simulink model "milestoneone_mdl_v2"  (R2025a)
settings: Solver=FixedStepAuto  StartTime=0.0  StopTime=10  FixedStep=1e-3  RelTol=1e-3  EnableMultiTasking=on
model workspace (MAT data in the model file):
  Var = 0
undefined symbols (not defined in the file): D0, D1, D10, D11, D12, D13, D2, D3, D4, D5, D6, D7, D8, D9, PTA0, PTA1, PTA2, PTB23, PTB9, PTC16, PTC17, PTC2, PTC3, PTC4, PTD0, PTD1, PTD2, PTD3
libraries: frdmk64flib x14
settings Model: ExtModeTrigDuration=5  Creator=alber  LastModifiedBy=ybakr
settings OptimizationCC: DefaultParameterBehavior=Inlined  EnhancedBackFolding=on  PassReuseOutputArgsAs=Individual arguments  ZeroExternalMemoryAtStartup=off  ZeroInternalMemoryAtStartup=off  MaxStackSize=64  OptimizeBlockOrder=speed  DifferentSizesBufferReuse=on  OptimizationCustomize=off  EfficientTunableParamExpr=on
settings DebuggingCC: ParameterTunabilityLossMsg=error
settings HardwareCC: ProdBitPerPointer=32.0  ProdBitPerSizeT=32.0  ProdBitPerPtrDiffT=32.0  ProdLargestAtomicInteger=Long  ProdLargestAtomicFloat=Double  ProdWordSize=32.0  ProdHWDeviceType=ARM Compatible->ARM Cortex
settings SFSimCC: MATLABDynamicMemAlloc=off
settings RTWCC: SystemTargetFile=ert.tlc  HardwareBoard=NXP FRDM-K64F  TLCOptions="-aInlineSetEventsForThisBaseRateFcn=TLC_FALSE -aSuppressMultiTaskScheduler=TLC_FALSE  -aRateBasedStepFcn=0"  TemplateMakefile=ert_default_tmf  Toolchain=GNU Tools for ARM Embedded Processors  Description=Embedded Coder
settings CodeAppCC: ForceParamTrailComments=on  IgnoreCustomStorageClasses=off  OperatorAnnotations=on  SimulinkDataObjDesc=on  SFDataObjDesc=on  InsertBlockDesc=on
settings ERTTargetCC: ExtModeTransport=4.0  ExtModeStaticAlloc=off  ExtModeMexFile=sendToCommService  ExtModeIntrfLevel=Level1

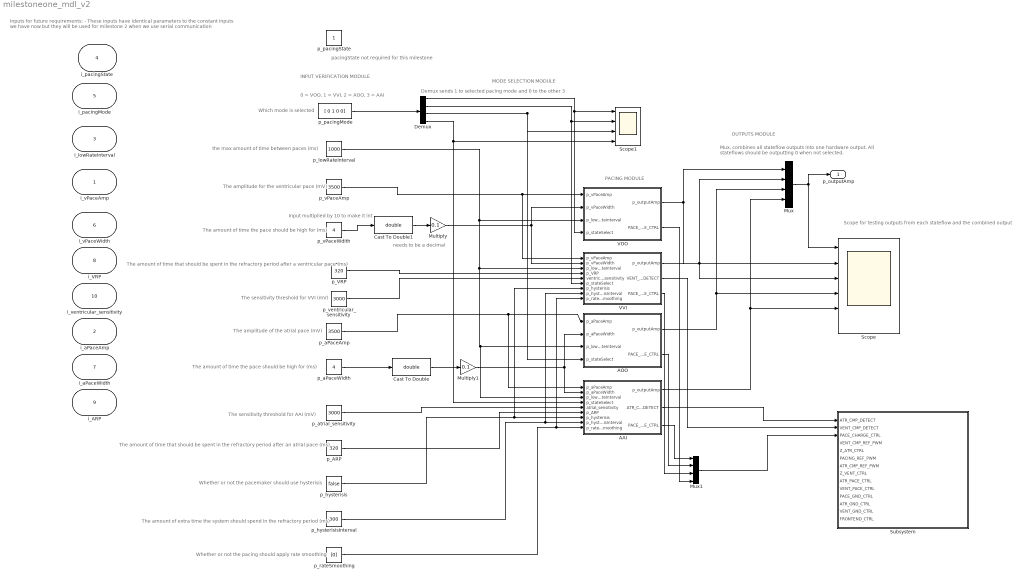
== system milestoneone_mdl_v2 ==
  note: The amount of extra time the system should spend in the refractory period (ms)
  note: Whether or not the pacemaker should use hysterisis
  note: Whether or not the pacing should apply rate smoothing
  note: The amplitude of the atrial pace (mV)
  note: The sensitivity threshold for VVI (mV)
  note: The amount of time that should be spent in the refractory period after a ventricular pace (ms)
  note: The amount of time the pace should be high for (ms)
  note: needs to be a decimal
  note: OUTPUTS MODULE
  note: PACING MODULE
  note: MODE SELECTION MODULE
  note: INPUT VERIFICATION MODULE
  note: The amplitude for the ventricular pace (mV)
  note: the max amount of time between paces (ms)
  note: Which mode is selected
  note: Inputs for future requirements:
      | - These inputs have identical parameters to the constant inputs we have now but they will be used for milestone 2 when we use serial communication
  note: pacingState not required for this milestone
  note: Demux sends 1 to selected pacing mode and 0 to the other 3
  note: Input multiplied by 10 to make it int
  note: 0 = VOO, 1 = VVI, 2 = AOO, 3 = AAI
  note: Scope for testing outputs from each stateflow and the combined output
  note: Mux, combines all stateflow outputs into one hardware output.
      | All stateflows should be outputting 0 when not selected.
  note: The amount of time the pace should be high for (ms)
  note: The sensitivity threshold for AAI (mV)
  note: The amount of time that should be spent in the refractory period after an atrial pace (ms)
  i_vPaceAmp : Inport  OutMin=[500]  OutMax=[7000]  OutDataTypeStr=uint16  Unit=mV  PortDimensions=1
  i_aPaceAmp : Inport  Port=2  OutMin=[500]  OutMax=[7000]  OutDataTypeStr=uint16  Unit=mV  PortDimensions=1
  i_lowRateInterval : Inport  Port=3  OutMin=[343]  OutMax=[2000]  OutDataTypeStr=uint16  Unit=Msec  PortDimensions=1
  i_pacingState : Inport  Port=4
  i_pacingMode : Inport  Port=5  OutDataTypeStr=uint8  PortDimensions=1
  i_vPaceWidth : Inport  Port=6  OutMin=1  OutMax=19  OutDataTypeStr=uint16  Unit=Msec  PortDimensions=1
  i_aPaceWidth : Inport  Port=7  OutMin=[1]  OutMax=[19]  OutDataTypeStr=uint16  Unit=Msec  PortDimensions=1
  i_VRP : Inport  Port=8  OutMin=[150]  OutMax=[500]  OutDataTypeStr=uint16  Unit=Msec  PortDimensions=1
  i_ARP : Inport  Port=9  OutMin=[150]  OutMax=[500]  OutDataTypeStr=uint16  Unit=mSec  PortDimensions=1
  i_ventricular_sensitivity : Inport  Port=10  OutDataTypeStr=uint16  PortDimensions=1
  AAI : Stateflow chart  TreatAsAtomicUnit=on
      settings: PortSchema="{\"entries\":[{\"content\":{\"sides\":[{\"content\":{\"connectorIds\":[\"In6\",\"In1\",\"In2\",\"In3\",\"In4\",\"In5\",\"In7\",\"In8\",\"In9\"]},\"type\":\"ConnectorPlacement.EquallySpacedRectSide\",\"uuid\":\"cccc9f32-b255-4089-8202-5f4b6cf4849a\"},{\"content\":{\"connectorIds\":[\"Out1\",\"Out2\",\"Out3\"],\"side\":\"RIGHT\"},\"type\":\"ConnectorPlacement.EquallySpacedRectSide\",\"uuid\":\"983a4a60-3d5c-4e53-84aa-b68c0bc6099e\"},{\"content\":{\"side\":\"TOP\"},\"type\":\"ConnectorPlacement.EquallySpacedRectSide\",\"uuid\":\"2756b790-cbb9-4039-b4f9-91cb14419ddd\"}]},\"type\":\"ConnectorPlacement.EquallySpacedConnector\",\"uuid\":\"1ccddf37-9dbc-46c0-8904-a3b9c6a38aa8\"}],\"packageUris\":[\"http://schema.mathworks.com/mf0/Connector/R2020b\"],\"version\":\"1.0\"}"
  AOO : Stateflow chart  TreatAsAtomicUnit=on
  Cast To Double : DataTypeConversion  OutDataTypeStr=double  SaturateOnIntegerOverflow=off  RndMeth=Floor
  Cast To Double1 : DataTypeConversion  OutDataTypeStr=double  SaturateOnIntegerOverflow=off  RndMeth=Floor
  Demux : Demux
  Multiply : Gain  Gain=0.1
  Multiply1 : Gain  Gain=0.1
  Mux : Mux
  Mux1 : Mux
  Scope : Scope  NumInputPorts=6
      settings: ActiveDisplayYMinimum=-128.4248  ActiveDisplayYMaximum=3655.0816
  Scope1 : Scope  NumInputPorts=4
      settings: ActiveDisplayYMinimum=-0.2183  ActiveDisplayYMaximum=1.8178
  Subsystem : Subsystem
  VOO : Stateflow chart  TreatAsAtomicUnit=on
  VVI : Stateflow chart  TreatAsAtomicUnit=on
  p_ARP : Constant  Value=320  OutMin=[150]  OutMax=[500]  OutDataTypeStr=uint16
  p_VRP : Constant  Value=320  OutMin=[150]  OutMax=[500]  OutDataTypeStr=uint16
  p_aPaceAmp : Constant  Value=3500  OutDataTypeStr=uint16
  p_aPaceWidth : Constant  Value=4  OutDataTypeStr=int16
  p_atrial_sensitivity : Constant  Value=3000  OutDataTypeStr=uint16
  p_hysterisis : Constant  Value=false  OutDataTypeStr=uint16
  p_hysterisisInterval : Constant  Value=300  OutDataTypeStr=uint16
  p_lowRateInterval : Constant  Value=1000  OutMin=[343]  OutMax=[2000]  OutDataTypeStr=uint16
  p_pacingMode : Constant  Value=[ 0 1 0 0]  OutDataTypeStr=uint8
  p_pacingState : Constant  OutDataTypeStr=uint8
  p_rateSmoothing : Constant  Value=[0]  OutDataTypeStr=uint16
  p_vPaceAmp : Constant  Value=3500  OutMin=[500]  OutMax=[7000]  OutDataTypeStr=uint16
  p_vPaceWdith : Constant  Value=4  OutMin=[1]  OutMax=[19]  OutDataTypeStr=int16
  p_ventricular_sensitivity : Constant  Value=3000  OutDataTypeStr=uint16
  p_outputAmp : Outport
  wires:
  VVI/1(p_outputAmp) -> Mux/2, Scope/3
  AOO/1(p_outputAmp) -> Mux/3, Scope/4
  Mux/1 -> p_outputAmp/1, Scope/1
  Multiply/1 -> VOO/2(p_vPaceWidth), VVI/2(p_vPaceWidth)
  Cast To Double1/1 -> Multiply/1
  Cast To Double/1 -> Multiply1/1
  Multiply1/1 -> AAI/1(p_aPaceWidth), AOO/2(p_aPaceWidth)
  Demux/1 -> Scope1/1, VOO/4(p_stateSelect)
  Demux/2 -> Scope1/2, VVI/6(p_stateSelect)
  Demux/3 -> Scope1/3, AOO/4(p_stateSelect)
  Demux/4 -> AAI/3(p_stateSelect), Scope1/4
  p_pacingMode/1 -> Demux/1
  p_aPaceWidth/1 -> Cast To Double/1
  p_aPaceAmp/1 -> AAI/6(p_aPaceAmp), AOO/1(p_aPaceAmp)
  p_lowRateInterval/1 -> AAI/2(p_lowRateInterval), AOO/3(p_lowRateInterval), VVI/3(p_lowRateInterval), VOO/3(p_lowRateInterval)
  p_vPaceAmp/1 -> VVI/1(p_vPaceAmp), VOO/1(p_vPaceAmp)
  p_vPaceWdith/1 -> Cast To Double1/1
  p_VRP/1 -> VVI/4(p_VRP)
  p_ventricular_sensitivity/1 -> VVI/5(ventricular_sensitivity)
  VOO/1(p_outputAmp) -> Scope/2, Mux/1
  p_ARP/1 -> AAI/5(p_ARP)
  p_atrial_sensitivity/1 -> AAI/4(atrial_sensitivity)
  p_hysterisis/1 -> VVI/7(p_hysterisis), AAI/7(p_hysterisis)
  p_hysterisisInterval/1 -> VVI/8(p_hysterisisInterval), AAI/8(p_hysterisisInterval)
  p_rateSmoothing/1 -> VVI/9(p_rateSmoothing), AAI/9(p_rateSmoothing)
  AAI/1(p_outputAmp) -> Mux/4, Scope/5
  AAI/2(ATR_CMP_DETECT) -> Subsystem/1("ATR_CMP_DETECT ")
  VVI/2(VENT_CMP_DETECT) -> Subsystem/2(VENT_CMP_DETECT)
  AAI/3(PACE_CHARGE_CTRL) -> Mux1/1
  Mux1/1 -> Subsystem/3(PACE_CHARGE_CTRL)
  AOO/2(PACE_CHARGE_CTRL) -> Mux1/2
  VVI/3(PACE_CHARGE_CTRL) -> Mux1/3
  VOO/2(PACE_CHARGE_CTRL) -> Mux1/4

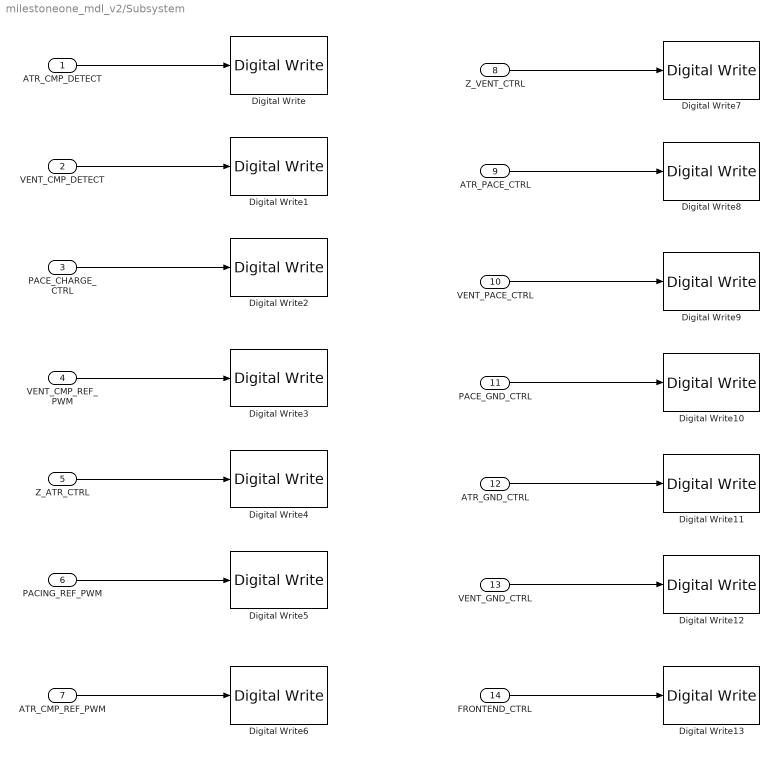
== system milestoneone_mdl_v2/Subsystem ==
  "ATR_CMP_DETECT " : Inport
  VENT_CMP_DETECT : Inport  Port=2
  PACE_CHARGE_CTRL : Inport  Port=3
  VENT_CMP_REF_PWM : Inport  Port=4
  Z_ATR_CTRL : Inport  Port=5
  PACING_REF_PWM : Inport  Port=6
  ATR_CMP_REF_PWM : Inport  Port=7
  Z_VENT_CTRL : Inport  Port=8
  ATR_PACE_CTRL : Inport  Port=9
  VENT_PACE_CTRL : Inport  Port=10
  PACE_GND_CTRL : Inport  Port=11
  ATR_GND_CTRL : Inport  Port=12
  VENT_GND_CTRL : Inport  Port=13
  FRONTEND_CTRL : Inport  Port=14
  Digital Write : frdmk64flib/Digital Write  Whichpin=PTC16 (D0)
  Digital Write1 : frdmk64flib/Digital Write  Whichpin=PTC17 (D1)
  Digital Write10 : frdmk64flib/Digital Write  Whichpin=PTD0 (D10)
  Digital Write11 : frdmk64flib/Digital Write  Whichpin=PTD2 (D11)
  Digital Write12 : frdmk64flib/Digital Write  Whichpin=PTD3 (D12)
  Digital Write13 : frdmk64flib/Digital Write  Whichpin=PTD1 (D13)
  Digital Write2 : frdmk64flib/Digital Write  Whichpin=PTB9 (D2)
  Digital Write3 : frdmk64flib/Digital Write  Whichpin=PTA1 (D3)
  Digital Write4 : frdmk64flib/Digital Write  Whichpin=PTB23 (D4)
  Digital Write5 : frdmk64flib/Digital Write  Whichpin=PTA2 (D5)
  Digital Write6 : frdmk64flib/Digital Write  Whichpin=PTC2 (D6)
  Digital Write7 : frdmk64flib/Digital Write  Whichpin=PTC3 (D7)
  Digital Write8 : frdmk64flib/Digital Write  Whichpin=PTA0 (D8)
  Digital Write9 : frdmk64flib/Digital Write  Whichpin=PTC4 (D9)
  wires:
  "ATR_CMP_DETECT "/1 -> Digital Write/1
  VENT_CMP_DETECT/1 -> Digital Write1/1
  PACE_CHARGE_CTRL/1 -> Digital Write2/1
  Z_ATR_CTRL/1 -> Digital Write4/1
  PACING_REF_PWM/1 -> Digital Write5/1
  VENT_CMP_REF_PWM/1 -> Digital Write3/1
  Z_VENT_CTRL/1 -> Digital Write7/1
  PACE_GND_CTRL/1 -> Digital Write10/1
  ATR_GND_CTRL/1 -> Digital Write11/1
  ATR_PACE_CTRL/1 -> Digital Write8/1
  VENT_PACE_CTRL/1 -> Digital Write9/1
  ATR_CMP_REF_PWM/1 -> Digital Write6/1
  VENT_GND_CTRL/1 -> Digital Write12/1
  FRONTEND_CTRL/1 -> Digital Write13/1

== stateflow chart milestoneone_mdl_v2/AOO ==
  note: Max total cycle time - time already elapsed this cycle
  note: AOO Pacing Mode
  note: Cycle through this state when AoO isn't selected
  state PACE
    entry:
    %Send out pace signal
    p_outputAmp = p_aPaceAmp;
    current_state = "AOO PACE"
    PACE_CHARGE_CTRL = 0;
    % Wait for the width of a pace
  state CHARGE
    entry:
    % Stop pacing, wait rest of cycle time
    p_outputAmp = 0;
    current_state = "AOO CHARGE"
    PACE_CHARGE_CTRL = 1;
  state INACTIVE
    % When state is not selected by input
  CHARGE -> PACE [order 2] : [after(p_lowRateInterval - p_aPaceWidth, msec)]
  (default) -> INACTIVE
  INACTIVE -> CHARGE [order 1] : [p_stateSelect == 1]
  CHARGE -> INACTIVE [order 1] : [p_stateSelect == 0]
  INACTIVE -> INACTIVE [order 2] : [p_stateSelect == 0]
  PACE -> CHARGE : after(p_aPaceWidth, msec)
  data: data local; p_outputAmp output uint16; p_aPaceAmp input uint16 =3500; p_aPaceWidth input double =0.4; p_lowRateInterval input uint16 =6000/low_rate_lim; p_stateSelect input uint8; current_state local string; PACE_CHARGE_CTRL output

== stateflow chart milestoneone_mdl_v2/VOO ==
  note: Total cycle time - time already elapsed this cycle
  note: VOO Pacing Mode
  state CHARGE
    entry:
    % Output 0V
    p_outputAmp = 0;
    current_state = "VOO CHARGE"
    PACE_CHARGE_CTRL = 1;
    % Rest time = total cycle time - pace width
  state PACE
    entry:
    % Output pace at specified amplitude
    p_outputAmp = p_vPaceAmp;
    current_state = "VOO PACE"
    PACE_CHARGE_CTRL = 0;
    % Wait so that the pace has the specified width
  state INACTIVE
    % Stateflow is inactive when not selected
  CHARGE -> PACE [order 2] : [after(p_lowRateInterval - p_vPaceWidth, msec)]
  (default) -> INACTIVE
  INACTIVE -> CHARGE [order 1] : [p_stateSelect == 1]
  CHARGE -> INACTIVE [order 1] : [p_stateSelect == 0]
  INACTIVE -> INACTIVE [order 2] : [p_stateSelect == 0]
  PACE -> CHARGE : after(p_vPaceWidth, msec)
  data: data local; p_outputAmp output uint16; p_vPaceAmp input uint16 =3500; p_vPaceWidth input double =0.4; p_lowRateInterval input uint16 =6000/low_rate_lim; p_stateSelect input uint8; current_state local string; PACE_CHARGE_CTRL output

== stateflow chart milestoneone_mdl_v2/AAI ==
  state PACING
    entry:
    state_out = "AAI PACING"
    p_outputAmp = p_aPaceAmp;
    end
  state WAIT
    entry:
    state_out = "AAI SENSING"
    entry:
    if ~isInitialized
    prevInterval = p_lowRateInterval;
    nextInterval = p_lowRateInterval;
    isInitialized = true;
    ATR_CMP_DETECT = 0;
    end
    PACE_CHARGE_CTRL = 0;
  state INACTIVE
  state REFRACTORY
    entry:
    state_out = "AAI REFRACTORY"
    f_waitInterval = p_ARP + p_hysterisis*p_hysterisisInterval;
    % Apply rate smoothing if enabled
    if ~p_rateSmoothing == 0
    delta = f_waitInterval - prevInterval;
    maxDelta = (p_rateSmoothing / 100) * prevInterval; %Percent Rate Smoothing
    if abs(delta) > maxDelta
    delta = maxDelta;
    end
    nextInterval = prevInterval + delta;
    prevInterval = nextInterval;
    end
    PACE_CHARGE_CTRL = 1;
  WAIT -> PACING [order 2] : [after(nextInterval,msec)]
  PACING -> REFRACTORY : [after(p_aPaceWidth, msec)]
  (default) -> INACTIVE
  WAIT -> REFRACTORY [order 3] : [p_aPaceAmp >= atrial_sensitivity]{ATR_CMP_DETECT = 1}
  INACTIVE -> WAIT [order 1] : [p_stateSelect == 1]
  WAIT -> INACTIVE [order 1] : [p_stateSelect == 0]
  INACTIVE -> INACTIVE [order 2] : [p_stateSelect == 0]
  REFRACTORY -> WAIT : [after(f_waitInterval,msec)]
  data: p_aPaceWidth input double =0.4; p_lowRateInterval input uint16 =6000/low_rate_lim; p_stateSelect input; atrial_sensitivity input; p_ARP input; p_aPaceAmp input; p_hysterisis input; p_hysterisisInterval input; p_rateSmoothing input; p_outputAmp output; delta local; f_waitInterval local; isInitialized local boolean =false; maxDelta local; nextInterval local; prevInterval local; state_out local string; ATR_CMP_DETECT output; PACE_CHARGE_CTRL output

== stateflow chart milestoneone_mdl_v2/VVI ==
  state PACING
    entry:
    current_state = "VVI PACING"
    % Generate pace
    p_outputAmp = p_vPaceAmp;
    PACE_CHARGE_CTRL = 0;
  note: VVI
  state REFRACTORY
    entry:
    current_state = "VVI REFRACTORY"
    % Stop generating pace
    p_outputAmp = 0;
    % Wait for a refractory period
    f_waitInterval = p_VRP + p_hysterisis*p_hysterisisInterval;
    if ~p_rateSmoothing == 0
    % Apply rate smoothing if enabled
    delta = f_waitInterval - prevInterval;
    maxDelta = (p_rateSmoothing / 100) * prevInterval; %Percent Rate Smoothing
    if abs(delta) > maxDelta
    delta = maxDelta;
    end
    nextInterval = prevInterval + delta;
    prevInterval = nextInterval;
    end
    PACE_CHARGE_CTRL = 1;
  note: Stateflow cycles in INACTIVE when not selected
  state SENSING
    entry:
    current_state = "VVI SENSING"
    if ~isInitialized
    prevInterval = p_lowRateInterval;
    nextInterval = p_lowRateInterval;
    isInitialized = true;
    VENT_CMP_DETECT = 1;
    end
    PACE_CHARGE_CTRL = 0;
    % If the input signal is higher than the
    % sensitivity threshold, wait for another
    % refractory period
    % If the low rate interval passes and no
    % signals higher than the threshold are
    % detected, send another pace
  state INACTIVE
    % When stateflow isn't selected
  PACING -> REFRACTORY : [after(p_vPaceWidth, msec)]
  (default) -> INACTIVE
  SENSING -> PACING [order 2] : [after(nextInterval, msec)]
  INACTIVE -> SENSING [order 1] : [p_stateSelect == 1]
  SENSING -> REFRACTORY [order 3] : [p_vPaceAmp >= ventricular_sensitivity]{VENT_CMP_DETECT = 1}
  SENSING -> INACTIVE [order 1] : [p_stateSelect == 0]
  REFRACTORY -> SENSING : [after(f_waitInterval, msec)]
  INACTIVE -> INACTIVE [order 2] : [p_stateSelect == 0]
  data: p_vPaceAmp input uint16 =3500; p_vPaceWidth input double =0.4; p_lowRateInterval input uint16 =6000/low_rate_lim; p_VRP input uint16; ventricular_sensitivity input uint16; p_outputAmp output uint16; p_stateSelect input uint8; current_state local string; p_hysterisis input; p_hysterisisInterval input; p_rateSmoothing input; delta local; f_waitInterval local; isInitialized local boolean =false; maxDelta local; nextInterval local; prevInterval local; VENT_CMP_DETECT output; PACE_CHARGE_CTRL output
